simulink model "power_3phPWM"  (Simulink 6.0)
settings: Solver=FixedStepDiscrete  SolverMode=SingleTasking  StartTime=0.0  StopTime=0.1  FixedStep=Ts  RelTol=1e-3
InitFcn:
  | Ts=1/60/3240;
undefined symbols (not defined in the file or in its folder): D1, Delta
libraries: powerlib x19, powerlib_extras x2
settings Model: Creator=patrice  LastModifiedBy=batserve  ExtModeTrigMode=oneshot  ExtModeArmWhenConnect=off  ExtModeAutoUpdateStatusClock=off
settings DataIOCC: LimitDataPoints=off  SignalLoggingName=sigsOut
settings OptimizationCC: BlockReduction=off  BooleanDataType=off
settings DebuggingCC: CheckExecutionContextPreStartOutputMsg=on  CheckExecutionContextRuntimeOutputMsg=on  SolverPrmCheckMsg=none
settings HardwareCC: TargetUnknown=on
settings RTWCC: TemplateMakefile=grt_unix.tmf

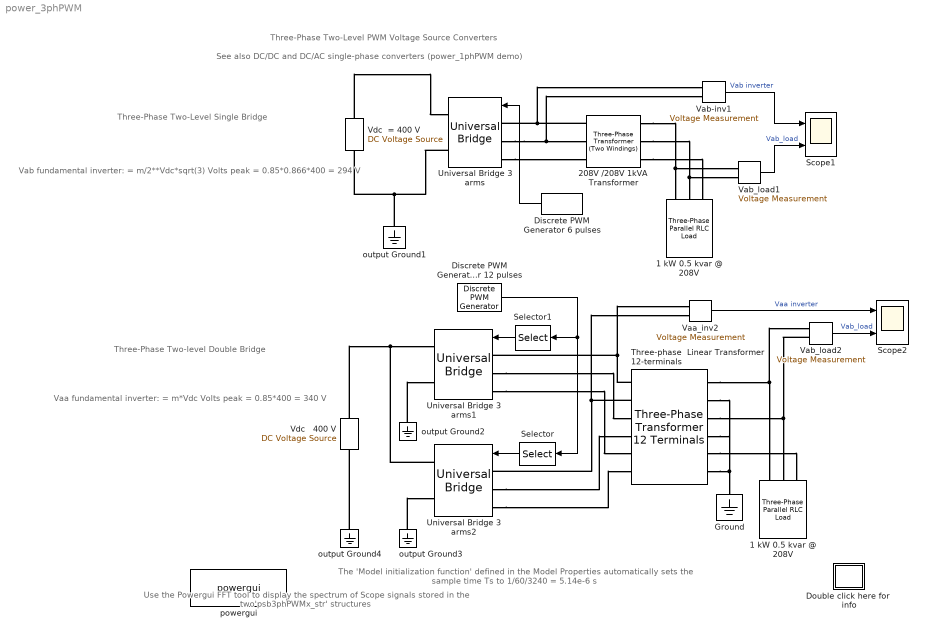
== system power_3phPWM ==
  note: Vaa fundamental inverter:
      | = m*Vdc Volts peak
      | = 0.85*400
      | = 340 V
  note: Three-Phase Two-Level PWM Voltage Source Converters
  note: See also DC/DC and DC/AC single-phase converters (power_1phPWM demo)
  note: Vab fundamental inverter:
      | = m/2**Vdc*sqrt(3) Volts peak
      | = 0.85*0.866*400
      | = 294 V
  note: Three-Phase Two-Level
      | Single Bridge
  note: Three-Phase Two-level
      | Double Bridge
  note: Use the Powergui FFT tool to display the
      | spectrum of Scope signals stored in the
      | two'psb3phPWMx_str' structures
  note: The 'Model  initialization function' defined in the
      | Model Properties automatically sets the sample time Ts
      | to 1/60/3240 = 5.14e-6 s
  1 kW 0.5 kvar @ 208V : powerlib/Elements/Three-Phase Parallel RLC Load  Orientation=down  PhysicalDomain=powersysdomain  SubClassName=unknown  LeftPortType=p1  RightPortType=p1  LConnTagsString=A|B|C  Configuration=Y (grounded)  NominalVoltage=208  NominalFrequency=60  ActivePower=1000  InductivePower=0  CapacitivePower=500  Measurements=None
  "1 kW 0.5 kvar @ 208V " : powerlib/Elements/Three-Phase Parallel RLC Load  Orientation=down  PhysicalDomain=powersysdomain  SubClassName=unknown  LeftPortType=p1  RightPortType=p1  LConnTagsString=A|B|C  Configuration=Y (grounded)  NominalVoltage=208  NominalFrequency=60  ActivePower=1000  InductivePower=0  CapacitivePower=500  Measurements=None
  208V /208V 1kVA Transformer : powerlib/Elements/Three-Phase Transformer (Two Windings)  NominalPower=[ 1000 , 60 ]  Winding1Connection=Delta (D1)  Winding1=[ 208 , 0.002 , 0.04 ]  Winding2Connection=Yg  Winding2=[ 208 , 0.002 , 0.04 ]  SetSaturation=off  Rm=200  Lm=200  Saturation="[ 0,0  ;  0.005,1.2  ;  1.0,1.4 ]"  Hysteresis=off  DataFile='hysteresis'  SetInitialFlux=off  InitialFluxes=[ 0.8 , -0.8 , 0.7 ]  Measurements=None  TransfoNumber=0
  Discrete PWM Generator 12 pulses : powerlib_extras/Discrete  Control Blocks/Discrete PWM Generator  GeneratorMode="Double 3-arm  bridges (12 pulses)"  Fc=1080  Ts=Ts  Internal=on  mIndex=0.85  Freq=60  Phase=0
  Discrete PWM Generator 6 pulses : powerlib_extras/Discrete  Control Blocks/Discrete PWM Generator  Orientation=left  GeneratorMode="3-arm  bridge (6 pulses)"  Fc=1080  Ts=Ts  Internal=on  mIndex=0.85  Freq=60  Phase=0
  Double click here for  info : Subsystem
      mask Display: disp('?')
  Ground : powerlib/Elements/Ground  Orientation=down  PhysicalDomain=powersysdomain  SubClassName=unknown  LeftPortType=p1  RightPortType=p1  LConnTagsString=a
  Scope1 : Scope  NumInputPorts=2
      settings: TimeRange=0.1  YMin=-500~-400  YMax=500~500  SaveName=psb3phPWM1_str  MaxDataPoints=500000
  Scope2 : Scope  NumInputPorts=2
      settings: TimeRange=0.1  YMin=-500~-300  YMax=500~400  SaveName=psb3phPWM2_str  MaxDataPoints=500000
  Selector : Selector  Orientation=left  Elements=7:12  InputPortWidth=12
  Selector1 : Selector  Orientation=left  Elements=1:6  InputPortWidth=12
  "Three-phase  Linear Transformer 12-terminals " : powerlib/Elements/Three-Phase Transformer 12 Terminals  RatedPower=[ 1000 60 ]  Winding1="[ 240  0.002  0.04 ]"  Winding2=[ 208/sqrt(3) 0.002 0.04]  RmXm=[ 200 200 ]
      settings: AttributesFormatString=\n
  Universal Bridge 3 arms : powerlib/Power Electronics/Universal Bridge  Orientation=left  Arms=3  SnubberResistance=10000  SnubberCapacitance=inf  Device=IGBT / Diodes  Ron=1e-4  Lon=0  ForwardVoltages="[  1  1  ]"  ForwardVoltage=.8  GTOparameters=[ 10e-6 , 20e-6 ]  IGBTparameters=[ 1e-6 , 2e-6 ]  Measurements=None
  Universal Bridge 3 arms1 : powerlib/Power Electronics/Universal Bridge  Orientation=left  Arms=3  SnubberResistance=10000  SnubberCapacitance=inf  Device=IGBT / Diodes  Ron=1e-4  Lon=0  ForwardVoltages="[  1  1  ]"  ForwardVoltage=.8  GTOparameters=[ 10e-6 , 20e-6 ]  IGBTparameters=[ 1e-6 , 2e-6 ]  Measurements=None
  Universal Bridge 3 arms2 : powerlib/Power Electronics/Universal Bridge  Orientation=left  Arms=3  SnubberResistance=10000  SnubberCapacitance=inf  Device=IGBT / Diodes  Ron=1e-4  Lon=0  ForwardVoltages="[  1  1  ]"  ForwardVoltage=.8  GTOparameters=[ 10e-6 , 20e-6 ]  IGBTparameters=[ 1e-6 , 2e-6 ]  Measurements=None
  Vaa_inv2 : powerlib/Measurements/Voltage Measurement  Tag=PoWeRsYsTeMmEaSuReMeNt  PhasorSimulation=off  OutputType=Magnitude  PSBequivalent=0
  Vab-inv1 : powerlib/Measurements/Voltage Measurement  Tag=PoWeRsYsTeMmEaSuReMeNt  PhasorSimulation=off  OutputType=Magnitude  PSBequivalent=0
  Vab_load1 : powerlib/Measurements/Voltage Measurement  Tag=PoWeRsYsTeMmEaSuReMeNt  PhasorSimulation=off  OutputType=Magnitude  PSBequivalent=0
  Vab_load2 : powerlib/Measurements/Voltage Measurement  Tag=PoWeRsYsTeMmEaSuReMeNt  PhasorSimulation=off  OutputType=Magnitude  PSBequivalent=0
  "Vdc   400 V " : powerlib/Electrical Sources/DC Voltage Source  Description=source block  Orientation=up  Amplitude=400  Measurements=None
      settings: AttributesFormatString=\n
  Vdc  = 400 V : powerlib/Electrical Sources/DC Voltage Source  Description=source block  Orientation=up  Amplitude=400  Measurements=None
      settings: AttributesFormatString=\n
  output Ground{1..4} (4 alike) : powerlib/Elements/Ground  Orientation=down  PhysicalDomain=powersysdomain  SubClassName=unknown  LeftPortType=p1  RightPortType=p1  LConnTagsString=a
  powergui : powerlib/powergui  Priority=2  Frange=[0:2:500]  Ylog=off  Xlog=off  save=off  variable=ZData  structure=psb3phPWM1_str  ZoomFFT=on  StartTime=0.1 - 2/60  cycles=2  DisplayStyle=off  fundamental=60  FreqAxis=off  MaxFrequency=5000  frequencyindice=1  frequencyindicesteady=1  RmsSteady=1  display=off  Ts=Ts  methode=off  frequency=60  echomessages=on
  wires:
  Discrete PWM Generator 6 pulses/1 -> Universal Bridge 3 arms/1
  Vab_load1/1 -> Scope1/2  "Vab_load"
  Vab-inv1/1 -> Scope1/1  "Vab inverter"
  Selector/1 -> Universal Bridge 3 arms2/1
  Vaa_inv2/1 -> Scope2/1  "Vaa inverter"
  Vab_load2/1 -> Scope2/2  "Vab_load"
  Selector1/1 -> Universal Bridge 3 arms1/1
  Discrete PWM Generator 12 pulses/1 -> Selector1/1, Selector/1
  connections:
  Universal Bridge 3 arms/LConn2 -- Vab-inv1/LConn2 -- 208V /208V 1kVA Transformer/LConn2
  Universal Bridge 3 arms/LConn3 -- 208V /208V 1kVA Transformer/LConn3
  208V /208V 1kVA Transformer/RConn3 -- 1 kW 0.5 kvar @ 208V/LConn3
  208V /208V 1kVA Transformer/RConn1 -- 1 kW 0.5 kvar @ 208V/LConn1 -- Vab_load1/LConn1
  208V /208V 1kVA Transformer/RConn2 -- 1 kW 0.5 kvar @ 208V/LConn2 -- Vab_load1/LConn2
  output Ground1/LConn1 -- Vdc  = 400 V/LConn1 -- Universal Bridge 3 arms/RConn2
  Vdc  = 400 V/RConn1 -- Universal Bridge 3 arms/RConn1
  208V /208V 1kVA Transformer/LConn1 -- Universal Bridge 3 arms/LConn1 -- Vab-inv1/LConn1
  output Ground2/LConn1 -- Universal Bridge 3 arms1/RConn2
  output Ground3/LConn1 -- Universal Bridge 3 arms2/RConn2
  output Ground4/LConn1 -- "Vdc   400 V "/LConn1
  "Three-phase  Linear Transformer 12-terminals "/LConn1 -- Universal Bridge 3 arms1/LConn1 -- Vaa_inv2/LConn1
  Universal Bridge 3 arms1/LConn2 -- "Three-phase  Linear Transformer 12-terminals "/LConn3
  Universal Bridge 3 arms1/LConn3 -- "Three-phase  Linear Transformer 12-terminals "/LConn5
  "Vdc   400 V "/RConn1 -- Universal Bridge 3 arms1/RConn1 -- Universal Bridge 3 arms2/RConn1
  "Three-phase  Linear Transformer 12-terminals "/LConn2 -- Universal Bridge 3 arms2/LConn1 -- Vaa_inv2/LConn2
  Universal Bridge 3 arms2/LConn2 -- "Three-phase  Linear Transformer 12-terminals "/LConn4
  Universal Bridge 3 arms2/LConn3 -- "Three-phase  Linear Transformer 12-terminals "/LConn6
  Vab_load2/LConn2 -- "1 kW 0.5 kvar @ 208V "/LConn2 -- "Three-phase  Linear Transformer 12-terminals "/RConn3
  "Three-phase  Linear Transformer 12-terminals "/RConn1 -- "1 kW 0.5 kvar @ 208V "/LConn1 -- Vab_load2/LConn1
  "Three-phase  Linear Transformer 12-terminals "/RConn2 -- "Three-phase  Linear Transformer 12-terminals "/RConn4 -- Ground/LConn1 -- "Three-phase  Linear Transformer 12-terminals "/RConn6
  "Three-phase  Linear Transformer 12-terminals "/RConn5 -- "1 kW 0.5 kvar @ 208V "/LConn3

== system power_3phPWM/Double click here for  info ==
  note: G. Sybille and P. Giroux (Hydro-Quebec)
  note: Demonstration
  note: Circuit Description
  note: This demonstration illustrates use of the Universal Bridge and
      | Discrete PWM Pulse Generator blocks. It also demonstrates
      | harmonic analysis of PWM waveforms using the Powergui/FFT tool.
  note: The system consists of two independent circuits illustrating two three-phase two-level PWM voltage source inverters.
      | Each  inverter feeds an AC load (1 kW, 500 var 60Hz @ 208V rms) through a three-phase transformer.
      | Both converters are controlled in open loop with the Discrete PWM Generator block available in the Extras/Discrete Control Blocks library.
      | The two circuits use the same DC voltage (Vdc = 400V), carrier frequency (1080 Hz), modulation index (m = 0.85) and generated frequency (f = 60 Hz).
      | Harmonic filtering is performed by the transformer leakage inductance (8%) and load capacitance (500 var).
      |
      | The two circuits are:
      |
      | 1. Three-phase,  two-level converter (one three-arm bridge; six-switches)
      | 2. Three-phase,  two-level converter (two three-arm bridge; twelve-switches in H configuration)
      |
      | In order to allow further signal processing, signals displayed on the two Scope blocks (sampled at simulation sampling rate of 3240 samples/ cycle)
      | are stored in two  variables named 'psb3phPWM1_str' and 'psb3phPWM2_str'  (structures with time) .
  note: Run the simulation and observe the following two waveforms on the Scope blocks:
      | Voltage generated by the PWM inverter (trace 1), load voltage (trace 2)
      |
      | Once the  simulation is completed, open the Powergui and select  'FFT Analysis' to display the 0-5000 Hz frequency spectrum of signals saved
      | in the two 'psb3phPWMx_str' structures. The FFT will be performed on  a 2-cycle window starting at t = 0.1 - 2/60 (last 2 cycles of recording).
      | For each circuit selelect Input labeled 'Vaa inverter'  or 'Vab inveter'. Click on Display and observe the frequency spectrum of last 2 cycles.
      |
      | The fundamental component of  V inverter is displayed above the spectrum window.
      | Compare the magnitude of the fundamental of the inverter voltage with the theoretical values given in the  circuit.
      |
      | Compare also the harmonic contents in the inverter voltage for the two-switch and four-switch DC/AC inverters.
      | For the six-switch inverter,  the first harmonics  occur around the carrier frequency (1080 Hz +- k*60Hz)
      | whereas for the twelve-switch inverter harmonics are lower and appear at double of carrier frequency.
      | As a result, the load voltage is "cleaner" for the twelve-switch inverter.
      | If you now perform a FFT on the signal Vab_load you will notice that the THD is 4.1% for the six-switch inverter as
      | compared to only 2.1% for the twelve-switch inverter.
